simulink model "globos_sim"  (R2022b)
settings: Solver=FixedStepAuto  StartTime=0.0  StopTime=60.0  FixedStep=0.1  RelTol=1e-3
values from neighbouring files (symbols this model uses):
  B1 = 0.1    [globos.m]
  force = 0.02    [globos.m]
  force_time = 3    [globos.m]
  K1 = 0.4    [globos.m]
  K2 = 0.3    [globos.m]
  M1 = 0.25    [globos.m]
  M2 = 0.1    [globos.m]
settings Model: Creator=Fran  LastModifiedBy=Fran

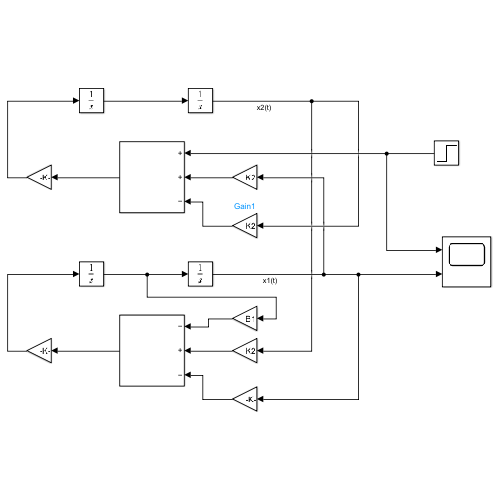
[thumbnail: Simulink's stored preview of the top-level diagram]
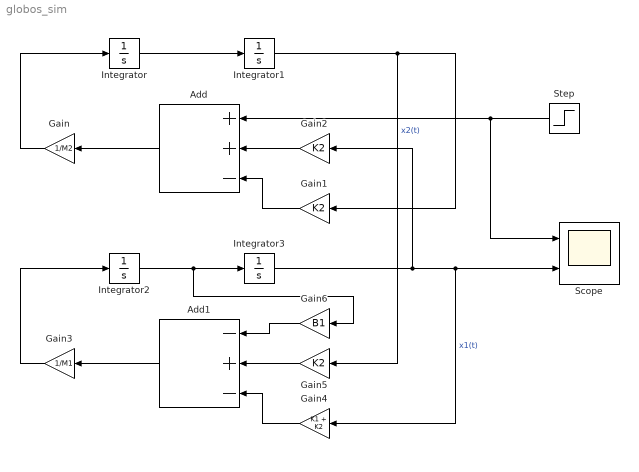
== system globos_sim ==
  Add : Sum  Inputs=++-
  Add1 : Sum  Inputs=-+-
  Gain : Gain  Gain=1/M2
  Gain1 : Gain  Gain=K2
  Gain2 : Gain  Gain=K2
  Gain3 : Gain  Gain=1/M1
  Gain4 : Gain  Gain=K1 + K2
  Gain5 : Gain  Gain=K2
  Gain6 : Gain  Gain=B1
  Integrator{,1..3} (4 alike) : Integrator
  Scope : Scope  NumInputPorts=2
  Step : Step  Time=force_time  Before=force  SampleTime=0
  wires:
  Integrator/1 -> Integrator1/1
  Gain/1 -> Integrator/1
  Add/1 -> Gain/1
  Gain1/1 -> Add/3
  Gain2/1 -> Add/2
  Integrator1/1 -> Gain5/1, Gain1/1  "x2(t)"
  Step/1 -> Scope/1, Add/1
  Integrator3/1 -> Gain2/1, Scope/2, Gain4/1  "x1(t)"
  Gain5/1 -> Add1/2
  Gain4/1 -> Add1/3
  Add1/1 -> Gain3/1
  Gain3/1 -> Integrator2/1
  Integrator2/1 -> Gain6/1, Integrator3/1
  Gain6/1 -> Add1/1
